simulink model "controle_atitude3"  (R2021b)
settings: Solver=ode45  StartTime=0.0  StopTime=100  MaxStep=0.4  RelTol=1e-3
values from neighbouring files (symbols this model uses):
  J = [0.00216966666667  0  0; 0  0.00216966666667  0; 0  0  0.00216966666667]    [parametros.mat]    (also in parametros2.mat)
  Jr = 3e-06    [parametros.mat]    (also in parametros2.mat)
  Jw = 0.0015    [parametros.mat]    (also in parametros2.mat)
  Ke = 0.000922    [parametros.mat]    (also in parametros2.mat)
  Km = 0.0264    [parametros.mat]    (also in parametros2.mat)
  Kt = 0.0088    [parametros.mat]    (also in parametros2.mat)
  L_a = 0.48    [parametros.mat]    (also in parametros2.mat)
  R_a = 7    [parametros.mat]    (also in parametros2.mat)
undefined symbols (not defined in the file or in its folder): K_lqr
libraries: aerolibutil x3, sharedutil x3, sharedtransform x2
settings Model: Creator=JRRL  LastModifiedBy=JRRL

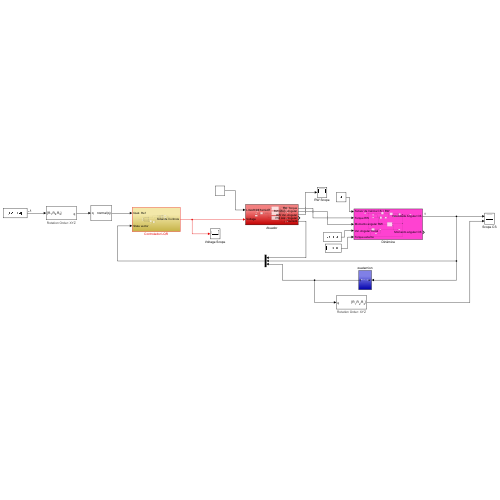
[thumbnail: Simulink's stored preview of the top-level diagram]
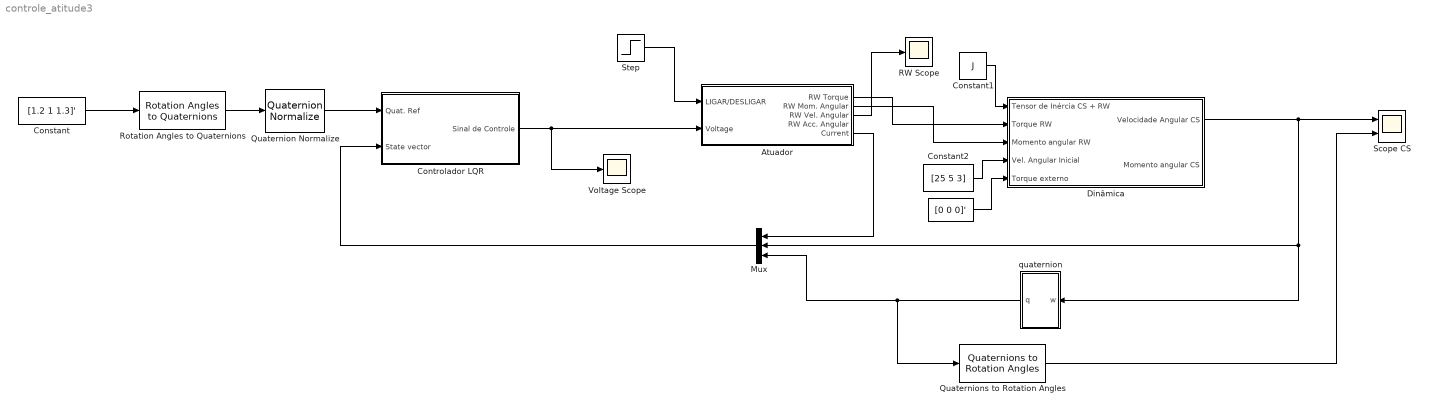
== system controle_atitude3 ==
  " " : Constant  Value=[0 0 0]'
  Atuador : Subsystem
  Constant : Constant  Value=[1.2 1 1.3]'
  Constant1 : Constant  Value=J
  Constant2 : Constant  Value=[25 5 3]
  Controlador LQR : Subsystem
  Dinâmica : Subsystem
  Mux : Mux  Inputs=3
  Quaternion Normalize : sharedutil/Quaternion Normalize  aMode=aMode
      settings: SourceProductBaseCode=AE,PW,DR,MT,UV,VE
  Quaternions to Rotation Angles : sharedtransform/Quaternions to Rotation Angles  rotationOrder=XYZ  aMode=aMode
      settings: SourceProductBaseCode=AE,PW,DR,MT,UV,VE
  RW Scope : Scope
  Rotation Angles to Quaternions : sharedtransform/Rotation Angles to Quaternions  rotationOrder=XYZ  aMode=aMode
      settings: SourceProductBaseCode=AE,PW,DR,MT,UV,VE
  Scope CS : Scope  NumInputPorts=2
  Step : Step  Time=100  Before=1  SampleTime=0
  Voltage Scope : Scope
  quaternion : Subsystem
  wires:
  Constant1/1 -> Dinâmica/1(Tensor de Inércia CS + RW)
  Dinâmica/1(Velocidade Angular CS) -> Scope CS/1, quaternion/1(w), Mux/2
  Atuador/2(RW Mom. Angular) -> Dinâmica/3(Momento angular RW)
  Constant2/1 -> Dinâmica/4(Vel. Angular Inicial)
  " "/1 -> Dinâmica/5(Torque externo)
  quaternion/1(q) -> Quaternions to Rotation Angles/1, Mux/3
  Atuador/1(RW Torque) -> Dinâmica/2(Torque RW)
  Step/1 -> Atuador/1(LIGAR/DESLIGAR)
  Constant/1 -> Rotation Angles to Quaternions/1
  Rotation Angles to Quaternions/1 -> Quaternion Normalize/1
  Quaternions to Rotation Angles/1 -> Scope CS/2
  Atuador/5(Current) -> Mux/1
  Mux/1 -> Controlador LQR/2(State vector)
  Quaternion Normalize/1 -> Controlador LQR/1(Quat. Ref)
  Atuador/3(RW Vel. Angular) -> RW Scope/1
  Controlador LQR/1(Sinal de Controle) -> Atuador/2(Voltage), Voltage Scope/1

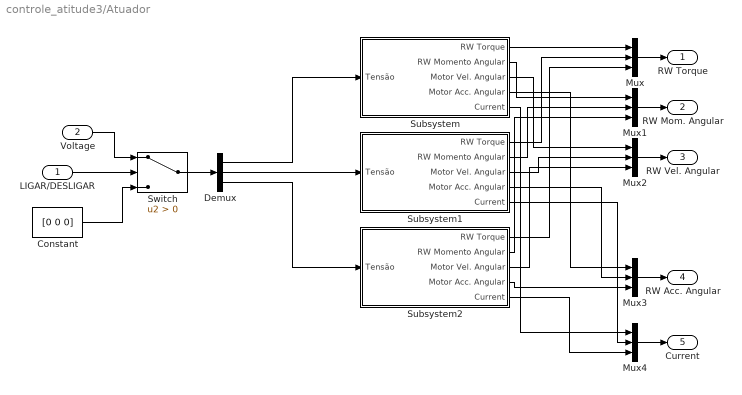
== system controle_atitude3/Atuador ==
  LIGAR/DESLIGAR : Inport
  Voltage : Inport  Port=2
  Constant : Constant  Value=[0 0 0]
  Demux : Demux  Outputs=3
  Mux{,1..4} (5 alike) : Mux  Inputs=3
  Subsystem : Subsystem
  Subsystem1 : Subsystem
  Subsystem2 : Subsystem
  Switch : Switch  Criteria=u2 > Threshold
  RW Torque : Outport
  RW Mom. Angular : Outport  Port=2
  RW Vel. Angular : Outport  Port=3
  RW Acc. Angular : Outport  Port=4
  Current : Outport  Port=5
  wires:
  Switch/1 -> Demux/1
  Demux/2 -> Subsystem1/1(Tensão)
  Demux/3 -> Subsystem2/1(Tensão)
  Subsystem1/1(RW Torque) -> Mux/2
  Subsystem2/1(RW Torque) -> Mux/3
  Mux/1 -> RW Torque/1
  Mux1/1 -> RW Mom. Angular/1
  Mux2/1 -> RW Vel. Angular/1
  Mux3/1 -> RW Acc. Angular/1
  LIGAR/DESLIGAR/1 -> Switch/2
  Voltage/1 -> Switch/1
  Constant/1 -> Switch/3
  Demux/1 -> Subsystem/1(Tensão)
  Subsystem/1(RW Torque) -> Mux/1
  Subsystem/2(RW Momento Angular) -> Mux1/1
  Subsystem/3(Motor Vel. Angular) -> Mux2/1
  Subsystem/4(Motor Acc. Angular) -> Mux3/1
  Mux4/1 -> Current/1
  Subsystem/5(Current) -> Mux4/1
  Subsystem1/2(RW Momento Angular) -> Mux1/2
  Subsystem2/2(RW Momento Angular) -> Mux1/3
  Subsystem1/3(Motor Vel. Angular) -> Mux2/2
  Subsystem2/3(Motor Vel. Angular) -> Mux2/3
  Subsystem1/4(Motor Acc. Angular) -> Mux3/2
  Subsystem2/4(Motor Acc. Angular) -> Mux3/3
  Subsystem1/5(Current) -> Mux4/2
  Subsystem2/5(Current) -> Mux4/3

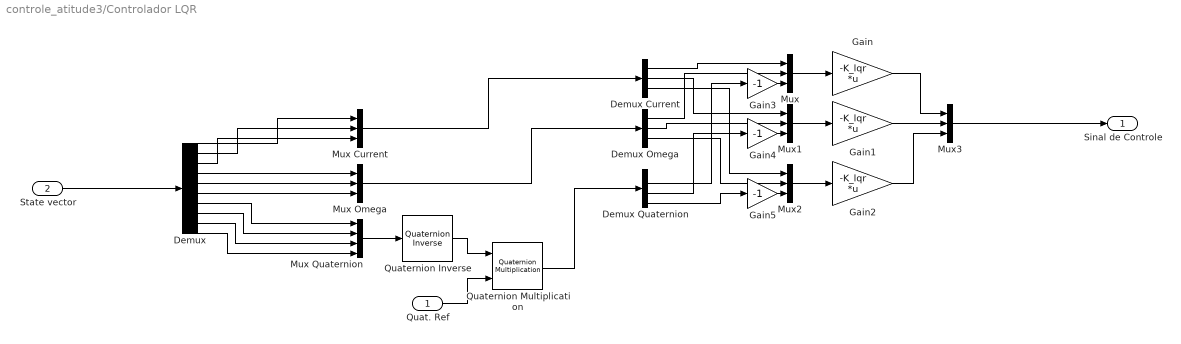
== system controle_atitude3/Controlador LQR ==
  Quat. Ref : Inport
  State vector : Inport  Port=2
  Demux : Demux  Outputs=10
  Demux Current : Demux  Outputs=3
  Demux Omega : Demux  Outputs=3
  Demux Quaternion : Demux
  Gain : Gain  Gain=-K_lqr  Multiplication=Matrix(K*u)
  Gain1 : Gain  Gain=-K_lqr  Multiplication=Matrix(K*u)
  Gain2 : Gain  Gain=-K_lqr  Multiplication=Matrix(K*u)
  Gain3 : Gain  Gain=-1
  Gain4 : Gain  Gain=-1
  Gain5 : Gain  Gain=-1
  Mux{,1..3} (4 alike) : Mux  Inputs=3
  Mux Current : Mux  Inputs=3
  Mux Omega : Mux  Inputs=3
  Mux Quaternion : Mux
  Quaternion Inverse : aerolibutil/Quaternion Inverse
  Quaternion Multiplication : aerolibutil/Quaternion Multiplication
  Sinal de Controle : Outport
  wires:
  Mux/1 -> Gain/1
  Mux1/1 -> Gain1/1
  Mux2/1 -> Gain2/1
  Gain1/1 -> Mux3/2
  Gain2/1 -> Mux3/3
  Gain3/1 -> Mux/3
  Gain4/1 -> Mux1/3
  Gain5/1 -> Mux2/3
  Gain/1 -> Mux3/1
  Mux3/1 -> Sinal de Controle/1
  Mux Quaternion/1 -> Quaternion Inverse/1
  Quat. Ref/1 -> Quaternion Multiplication/2
  Quaternion Inverse/1 -> Quaternion Multiplication/1
  Demux/7 -> Mux Quaternion/1
  Demux/8 -> Mux Quaternion/2
  Demux/9 -> Mux Quaternion/3
  Demux/10 -> Mux Quaternion/4
  Demux/1 -> Mux Current/1
  Demux/2 -> Mux Current/2
  Demux/3 -> Mux Current/3
  Demux/5 -> Mux Omega/2
  Demux/6 -> Mux Omega/3
  Demux/4 -> Mux Omega/1
  Quaternion Multiplication/1 -> Demux Quaternion/1
  Demux Quaternion/2 -> Gain3/1
  Demux Quaternion/3 -> Gain4/1
  Demux Quaternion/4 -> Gain5/1
  Mux Current/1 -> Demux Current/1
  Mux Omega/1 -> Demux Omega/1
  Demux Current/1 -> Mux/1
  Demux Current/2 -> Mux1/1
  Demux Current/3 -> Mux2/1
  Demux Omega/1 -> Mux/2
  Demux Omega/2 -> Mux1/2
  Demux Omega/3 -> Mux2/2
  State vector/1 -> Demux/1

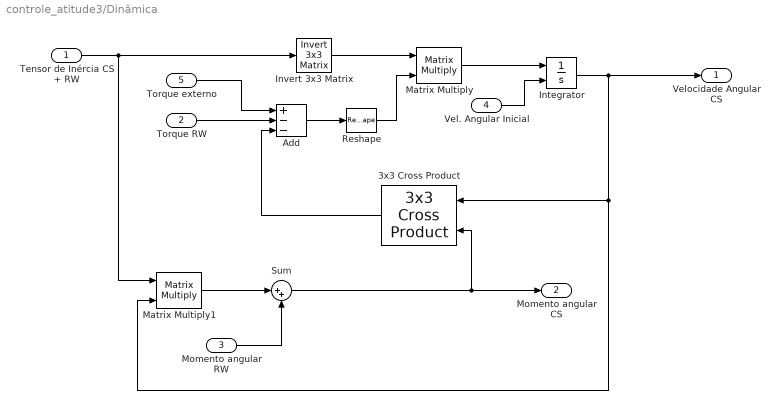
== system controle_atitude3/Dinâmica ==
  Tensor de Inércia CS + RW : Inport
  Torque RW : Inport  Port=2
  Momento angular RW : Inport  Port=3
  Vel. Angular Inicial : Inport  Port=4
  Torque externo : Inport  Port=5
  3x3 Cross Product : sharedutil/3x3 Cross Product  aMode=aMode
      settings: SourceProductBaseCode=AE,PW,DR,MT,UV,VE
  Add : Sum  Inputs=+--
  Integrator : Integrator  InitialConditionSource=external
  Invert 3x3 Matrix : aerolibutil/Invert  3x3 Matrix
  Matrix Multiply : Product  Multiplication=Matrix(*)
  Matrix Multiply1 : Product  Multiplication=Matrix(*)
  Reshape : Reshape  OutputDimensionality=Column vector (2-D)
  Sum : Sum  Inputs=|++
  Velocidade Angular CS : Outport
  Momento angular CS : Outport  Port=2
  wires:
  Sum/1 -> Momento angular CS/1, 3x3 Cross Product/2
  3x3 Cross Product/1 -> Add/3
  Invert 3x3 Matrix/1 -> Matrix Multiply/1
  Integrator/1 -> Velocidade Angular CS/1, Matrix Multiply1/2, 3x3 Cross Product/1
  Matrix Multiply/1 -> Integrator/1
  Momento angular RW/1 -> Sum/2
  Torque RW/1 -> Add/2
  Tensor de Inércia CS + RW/1 -> Matrix Multiply1/1, Invert 3x3 Matrix/1
  Torque externo/1 -> Add/1
  Vel. Angular Inicial/1 -> Integrator/2
  Add/1 -> Reshape/1
  Matrix Multiply1/1 -> Sum/1
  Reshape/1 -> Matrix Multiply/2

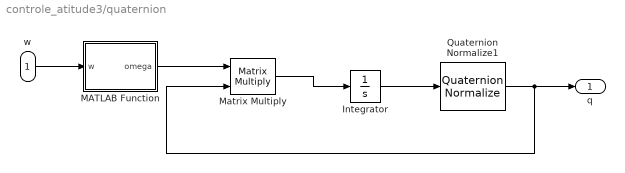
== system controle_atitude3/quaternion ==
  w : Inport
  Integrator : Integrator  InitialCondition=[1 0 0 0]
  MATLAB Function : MATLAB Function  TreatAsAtomicUnit=on
  Matrix Multiply : Product  Multiplication=Matrix(*)
  Quaternion Normalize1 : sharedutil/Quaternion Normalize  aMode=aMode
      settings: SourceProductBaseCode=AE,PW,DR,MT,UV,VE
  q : Outport
  wires:
  w/1 -> MATLAB Function/1(w)
  MATLAB Function/1(omega) -> Matrix Multiply/1
  Quaternion Normalize1/1 -> q/1, Matrix Multiply/2
  Matrix Multiply/1 -> Integrator/1
  Integrator/1 -> Quaternion Normalize1/1

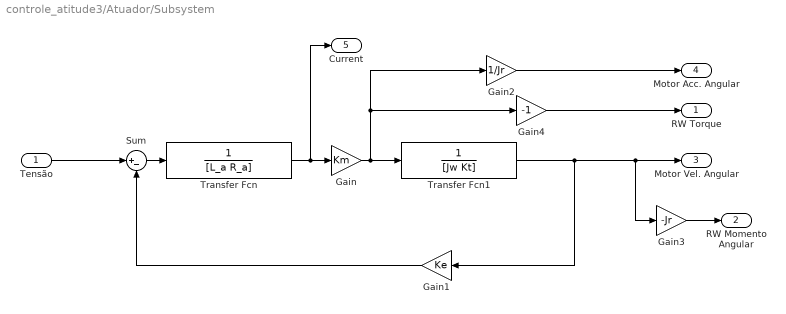
== system controle_atitude3/Atuador/Subsystem ==
  Tensão : Inport
  Gain : Gain  Gain=Km
  Gain1 : Gain  Gain=Ke
  Gain2 : Gain  Gain=1/Jr
  Gain3 : Gain  Gain=-Jr
  Gain4 : Gain  Gain=-1
  Sum : Sum  Inputs=|+-
  Transfer Fcn : TransferFcn  Denominator=[L_a R_a]
  Transfer Fcn1 : TransferFcn  Denominator=[Jw Kt]
  RW Torque : Outport
  RW Momento Angular : Outport  Port=2
  Motor Vel. Angular : Outport  Port=3
  Motor Acc. Angular : Outport  Port=4
  Current : Outport  Port=5
  wires:
  Gain/1 -> Transfer Fcn1/1, Gain4/1, Gain2/1
  Transfer Fcn/1 -> Current/1, Gain/1
  Gain2/1 -> Motor Acc. Angular/1
  Transfer Fcn1/1 -> Gain3/1, Motor Vel. Angular/1, Gain1/1
  Sum/1 -> Transfer Fcn/1
  Gain1/1 -> Sum/2
  Gain4/1 -> RW Torque/1
  Tensão/1 -> Sum/1
  Gain3/1 -> RW Momento Angular/1

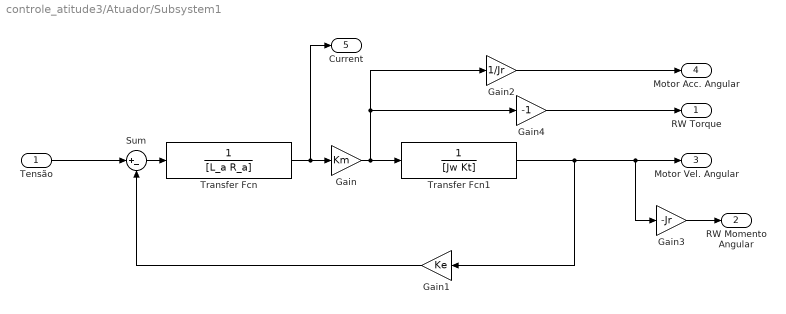
== system controle_atitude3/Atuador/Subsystem1 ==
  Tensão : Inport
  Gain : Gain  Gain=Km
  Gain1 : Gain  Gain=Ke
  Gain2 : Gain  Gain=1/Jr
  Gain3 : Gain  Gain=-Jr
  Gain4 : Gain  Gain=-1
  Sum : Sum  Inputs=|+-
  Transfer Fcn : TransferFcn  Denominator=[L_a R_a]
  Transfer Fcn1 : TransferFcn  Denominator=[Jw Kt]
  RW Torque : Outport
  RW Momento Angular : Outport  Port=2
  Motor Vel. Angular : Outport  Port=3
  Motor Acc. Angular : Outport  Port=4
  Current : Outport  Port=5
  wires:
  Gain/1 -> Transfer Fcn1/1, Gain4/1, Gain2/1
  Transfer Fcn/1 -> Current/1, Gain/1
  Gain2/1 -> Motor Acc. Angular/1
  Transfer Fcn1/1 -> Gain3/1, Motor Vel. Angular/1, Gain1/1
  Sum/1 -> Transfer Fcn/1
  Gain1/1 -> Sum/2
  Gain4/1 -> RW Torque/1
  Tensão/1 -> Sum/1
  Gain3/1 -> RW Momento Angular/1

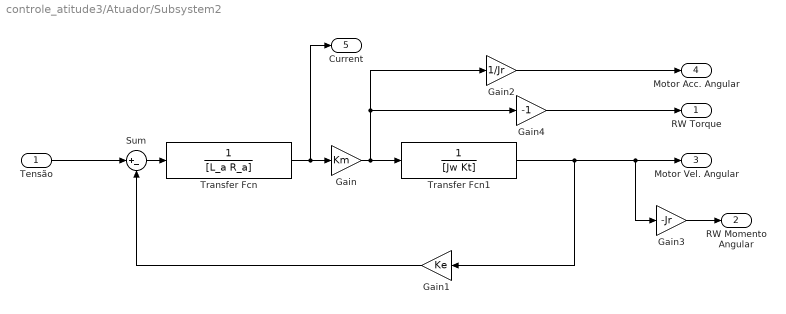
== system controle_atitude3/Atuador/Subsystem2 ==
  Tensão : Inport
  Gain : Gain  Gain=Km
  Gain1 : Gain  Gain=Ke
  Gain2 : Gain  Gain=1/Jr
  Gain3 : Gain  Gain=-Jr
  Gain4 : Gain  Gain=-1
  Sum : Sum  Inputs=|+-
  Transfer Fcn : TransferFcn  Denominator=[L_a R_a]
  Transfer Fcn1 : TransferFcn  Denominator=[Jw Kt]
  RW Torque : Outport
  RW Momento Angular : Outport  Port=2
  Motor Vel. Angular : Outport  Port=3
  Motor Acc. Angular : Outport  Port=4
  Current : Outport  Port=5
  wires:
  Gain/1 -> Transfer Fcn1/1, Gain4/1, Gain2/1
  Transfer Fcn/1 -> Current/1, Gain/1
  Gain2/1 -> Motor Acc. Angular/1
  Transfer Fcn1/1 -> Gain3/1, Motor Vel. Angular/1, Gain1/1
  Sum/1 -> Transfer Fcn/1
  Gain1/1 -> Sum/2
  Gain4/1 -> RW Torque/1
  Tensão/1 -> Sum/1
  Gain3/1 -> RW Momento Angular/1

== matlab function controle_atitude3/quaternion/MATLAB Function ==
  data: w input; omega output
function omega = fcn(w)
    wx = w(1);
    wy = w(2);
    wz = w(3);
    res = [0 -wx -wy -wz;wx 0 wz -wy;wy -wz 0 wx;wz wy -wx 0];
omega = res;
